simulink model "BEV_WHR"  (R2023a)
settings: Solver=ode23tb  StartTime=0.0  StopTime=20e3  MaxStep=1  RelTol=1e-3
values from neighbouring files (symbols this model uses):
  mass = 20e3    (= 20000)    [run_BEV_simulations.m]    (also in run_FCHEV_simulations.m)
libraries: component_lib x107, slpidlib x8
(part 1 of 2)
settings Model: Creator=maxjo  LastModifiedBy=maxjo
settings SolverCC: ZeroCrossControl=DisableAll

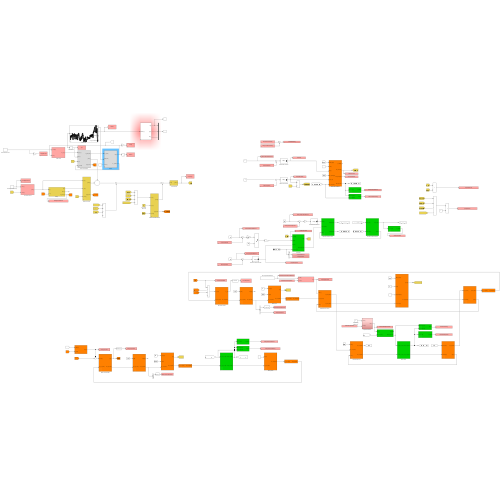
[thumbnail: Simulink's stored preview of the top-level diagram]
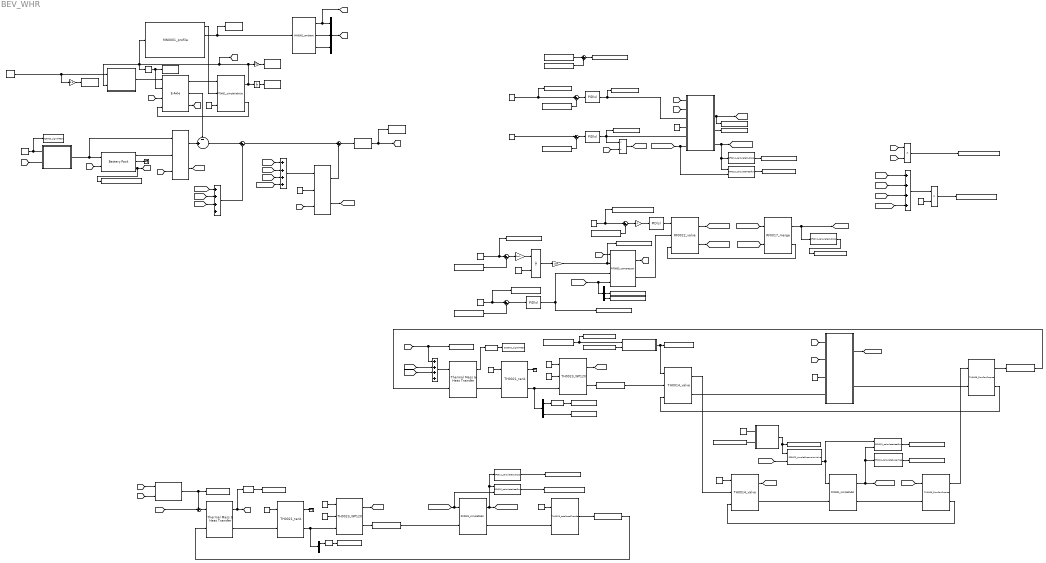
== system BEV_WHR ==
  Add{,1..3} (4 alike) : Sum  Inputs=++++
  Add Constant{,1..3} (4 alike) : Bias  Bias=-273.15  SaturateOnIntegerOverflow=off
  Battery : component_lib/Battery Pack  SOC_0=0.9  Nx=250  Ny=180
  Battery Heater : component_lib/Thermal Systems/TH0015_totalHeatTransfer  T_max=273+100  T_min=273
  Battery Thermal Mass : component_lib/Thermal Mass & Heat Transfer  n=100  d=10e-3  L=4  m=250 * 180 * 0.048  cp=1040  T_0=273 + 20
  Bus Voltage Control : Subsystem
  Bus Voltage Reference [V] : Constant  Value=700
  Cabin Airflow Controller : slpidlib/PID Controller  Controller=PID  Form=Parallel  TimeDomain=Continuous-time  UseExternalTs=off  SampleTime=-1  IntegratorMethod=Forward Euler  FilterMethod=Forward Euler  ControllerParametersSource=internal  P=1  I=1e-1  UseKiTs=off  D=0  N=100  UseFilter=on  TunerSelectOption=Transfer Function Based (PID Tuner App)  InitialConditionSource=internal  InitialConditionForIntegrator=0.5  InitialConditionForFilter=0  DifferentiatorICPrevScaledInput=0  ExternalReset=none  TrackingMode=off  Kt=1  LimitOutput=on  SatLimitsSource=internal  UpperSaturationLimit=1  LowerSaturationLimit=0  LinearizeAsGain=on  AntiWindupMode=clamping  Kb=1  LimitIntegrator=off  UpperIntegratorSaturationLimit=inf  LowerIntegratorSaturationLimit=-inf  POutMin=[]  POutMax=[]  IOutMin=[]  IOutMax=[]  DOutMin=[]  DOutMax=[]  NOutMin=[]  NOutMax=[]  SumOutMin=[]  SumOutMax=[]  SaturationOutMin=[]  SaturationOutMax=[]  PParamMin=[]  PParamMax=[]  IParamMin=[]  IParamMax=[]  DParamMin=[]  DParamMax=[]  NParamMin=[]  NParamMax=[]  KbParamMin=[]  KbParamMax=[]  KtParamMin=[]  KtParamMax=[]  KbOutMin=[]  KbOutMax=[]  KtOutMin=[]  KtOutMax=[]  IntegratorOutMin=[]  IntegratorOutMax=[]  FilterOutMin=[]  FilterOutMax=[]  SumI1OutMin=[]  SumI1OutMax=[]  SumI2OutMin=[]  SumI2OutMax=[]  SumI3OutMin=[]  SumI3OutMax=[]  SumI4OutMin=[]  SumI4OutMax=[]  SumDOutMin=[]  SumDOutMax=[]  DifferentiatorOutMin=[]  DifferentiatorOutMax=[]  FilterDiffOutCoefMin=[]  FilterDiffOutCoefMax=[]  ReciprocalOutMin=[]  ReciprocalOutMax=[]  SumDenOutMin=[]  SumDenOutMax=[]  SumNumOutMin=[]  SumNumOutMax=[]  DivideOutMin=[]  DivideOutMax=[]  UdiffTsProdOutMin=[]  UdiffTsProdOutMax=[]  NTsProdOutMin=[]  NTsProdOutMax=[]  UintegralTsProdOutMin=[]  UintegralTsProdOutMax=[]  UngainTsProdOutMin=[]  UngainTsProdOutMax=[]  ClampingZeroOutDataTypeStr=Inherit: Inherit via back propagation  ClampingZeroOutMin=[]  ClampingZeroOutMax=[]  FilterDenConstantOutDataTypeStr=Inherit: Inherit via back propagation  FilterDenConstantOutMin=[]  FilterDenConstantOutMax=[]  PCopyOutDataTypeStr=Inherit: Inherit via back propagation  PCopyOutMin=[]  PCopyOutMax=[]  NCopyOutDataTypeStr=Inherit: Inherit via back propagation  NCopyOutMin=[]  NCopyOutMax=[]  IntegratorContinuousStateAttributes=''  IntegratorStateMustResolveToSignalObject=off  IntegratorRTWStateStorageClass=Auto  FilterContinuousStateAttributes=''  FilterStateMustResolveToSignalObject=off  FilterRTWStateStorageClass=Auto  ParallelPVariant=InternalParameters  IdealPVariant=Disabled  IVariant=InternalParameters  DVariant=InternalParameters  IntegratorVariant=Continuous  SatVariant=Enabled  AWVariant=ContClampingParallel  PCopyVariant=Disabled  TRVariant=Disabled  FdbkBlocksVariant=Forward  IdealPFdbkVariant=Disabled  SatFdbkVariant=Disabled  DerivativeFilterVariant=ContFilter  NVariant=InternalParameters  NCopyVariant=Disabled  FilterICVariant=InternalICsFilter  IntegratorICVariant=InternalICs  ExternalResetVariant=Disabled  TRSumVariant=Passthrough  SumFdbkVariant=Disabled  SumVariant=Sum_PID  TsampFilterVariant=InternalTs  TsampNgainVariant=Passthrough  TsampIntegralVariant=Disabled_SignalSpec  ExternalSaturationOutDataTypeStr=Inherit: Same as second input
  Cabin with Condenser : Subsystem
  Chassi : component_lib/Powertrain/PT0001_simpleVehicle  m=mass  r_w=0.5  A_f=10  C_d=0.5  rho_air=1.225  c_r0=0.0060  c_r1=2.3e-7  gain=600  v0=75/3.6  x0=0
  Chiller Bypass Valve : component_lib/Thermal Systems/TH0014_valve  d=10e-2  dr=5e-2  C_d=0.9
  Compressor : component_lib/Thermal Systems/RF0003_compressor  V_disp=0.00017  N_ref=2000  t_c=1  W0=0
  Compressor Speed Controller : slpidlib/PID Controller  Controller=PID  Form=Parallel  TimeDomain=Continuous-time  UseExternalTs=off  SampleTime=-1  IntegratorMethod=Forward Euler  FilterMethod=Forward Euler  ControllerParametersSource=internal  P=1e2  I=1e1  UseKiTs=off  D=0  N=100  UseFilter=on  TunerSelectOption=Transfer Function Based (PID Tuner App)  InitialConditionSource=internal  InitialConditionForIntegrator=2000  InitialConditionForFilter=2000  DifferentiatorICPrevScaledInput=0  ExternalReset=none  TrackingMode=off  Kt=1  LimitOutput=on  SatLimitsSource=internal  UpperSaturationLimit=5000  LowerSaturationLimit=500  LinearizeAsGain=on  AntiWindupMode=clamping  Kb=1  LimitIntegrator=off  UpperIntegratorSaturationLimit=inf  LowerIntegratorSaturationLimit=-inf  POutMin=[]  POutMax=[]  IOutMin=[]  IOutMax=[]  DOutMin=[]  DOutMax=[]  NOutMin=[]  NOutMax=[]  SumOutMin=[]  SumOutMax=[]  SaturationOutMin=[]  SaturationOutMax=[]  PParamMin=[]  PParamMax=[]  IParamMin=[]  IParamMax=[]  DParamMin=[]  DParamMax=[]  NParamMin=[]  NParamMax=[]  KbParamMin=[]  KbParamMax=[]  KtParamMin=[]  KtParamMax=[]  KbOutMin=[]  KbOutMax=[]  KtOutMin=[]  KtOutMax=[]  IntegratorOutMin=[]  IntegratorOutMax=[]  FilterOutMin=[]  FilterOutMax=[]  SumI1OutMin=[]  SumI1OutMax=[]  SumI2OutMin=[]  SumI2OutMax=[]  SumI3OutMin=[]  SumI3OutMax=[]  SumI4OutMin=[]  SumI4OutMax=[]  SumDOutMin=[]  SumDOutMax=[]  DifferentiatorOutMin=[]  DifferentiatorOutMax=[]  FilterDiffOutCoefMin=[]  FilterDiffOutCoefMax=[]  ReciprocalOutMin=[]  ReciprocalOutMax=[]  SumDenOutMin=[]  SumDenOutMax=[]  SumNumOutMin=[]  SumNumOutMax=[]  DivideOutMin=[]  DivideOutMax=[]  UdiffTsProdOutMin=[]  UdiffTsProdOutMax=[]  NTsProdOutMin=[]  NTsProdOutMax=[]  UintegralTsProdOutMin=[]  UintegralTsProdOutMax=[]  UngainTsProdOutMin=[]  UngainTsProdOutMax=[]  ClampingZeroOutDataTypeStr=Inherit: Inherit via back propagation  ClampingZeroOutMin=[]  ClampingZeroOutMax=[]  FilterDenConstantOutDataTypeStr=Inherit: Inherit via back propagation  FilterDenConstantOutMin=[]  FilterDenConstantOutMax=[]  PCopyOutDataTypeStr=Inherit: Inherit via back propagation  PCopyOutMin=[]  PCopyOutMax=[]  NCopyOutDataTypeStr=Inherit: Inherit via back propagation  NCopyOutMin=[]  NCopyOutMax=[]  IntegratorContinuousStateAttributes=''  IntegratorStateMustResolveToSignalObject=off  IntegratorRTWStateStorageClass=Auto  FilterContinuousStateAttributes=''  FilterStateMustResolveToSignalObject=off  FilterRTWStateStorageClass=Auto  ParallelPVariant=InternalParameters  IdealPVariant=Disabled  IVariant=InternalParameters  DVariant=InternalParameters  IntegratorVariant=Continuous  SatVariant=Enabled  AWVariant=ContClampingParallel  PCopyVariant=Disabled  TRVariant=Disabled  FdbkBlocksVariant=Forward  IdealPFdbkVariant=Disabled  SatFdbkVariant=Disabled  DerivativeFilterVariant=ContFilter  NVariant=InternalParameters  NCopyVariant=Disabled  FilterICVariant=InternalICsFilter  IntegratorICVariant=InternalICs  ExternalResetVariant=Disabled  TRSumVariant=Passthrough  SumFdbkVariant=Disabled  SumVariant=Sum_PID  TsampFilterVariant=InternalTs  TsampNgainVariant=Passthrough  TsampIntegralVariant=Disabled_SignalSpec  ExternalSaturationOutDataTypeStr=Inherit: Same as second input
  Condenser Valve Controller : slpidlib/PID Controller  Controller=PID  Form=Parallel  TimeDomain=Continuous-time  UseExternalTs=off  SampleTime=-1  IntegratorMethod=Forward Euler  FilterMethod=Forward Euler  ControllerParametersSource=internal  P=1e-1  I=1e-2  UseKiTs=off  D=0  N=100  UseFilter=on  TunerSelectOption=Transfer Function Based (PID Tuner App)  InitialConditionSource=internal  InitialConditionForIntegrator=0.5  InitialConditionForFilter=0.5  DifferentiatorICPrevScaledInput=0  ExternalReset=none  TrackingMode=off  Kt=1  LimitOutput=on  SatLimitsSource=internal  UpperSaturationLimit=1  LowerSaturationLimit=0  LinearizeAsGain=on  AntiWindupMode=clamping  Kb=1  LimitIntegrator=off  UpperIntegratorSaturationLimit=inf  LowerIntegratorSaturationLimit=-inf  POutMin=[]  POutMax=[]  IOutMin=[]  IOutMax=[]  DOutMin=[]  DOutMax=[]  NOutMin=[]  NOutMax=[]  SumOutMin=[]  SumOutMax=[]  SaturationOutMin=[]  SaturationOutMax=[]  PParamMin=[]  PParamMax=[]  IParamMin=[]  IParamMax=[]  DParamMin=[]  DParamMax=[]  NParamMin=[]  NParamMax=[]  KbParamMin=[]  KbParamMax=[]  KtParamMin=[]  KtParamMax=[]  KbOutMin=[]  KbOutMax=[]  KtOutMin=[]  KtOutMax=[]  IntegratorOutMin=[]  IntegratorOutMax=[]  FilterOutMin=[]  FilterOutMax=[]  SumI1OutMin=[]  SumI1OutMax=[]  SumI2OutMin=[]  SumI2OutMax=[]  SumI3OutMin=[]  SumI3OutMax=[]  SumI4OutMin=[]  SumI4OutMax=[]  SumDOutMin=[]  SumDOutMax=[]  DifferentiatorOutMin=[]  DifferentiatorOutMax=[]  FilterDiffOutCoefMin=[]  FilterDiffOutCoefMax=[]  ReciprocalOutMin=[]  ReciprocalOutMax=[]  SumDenOutMin=[]  SumDenOutMax=[]  SumNumOutMin=[]  SumNumOutMax=[]  DivideOutMin=[]  DivideOutMax=[]  UdiffTsProdOutMin=[]  UdiffTsProdOutMax=[]  NTsProdOutMin=[]  NTsProdOutMax=[]  UintegralTsProdOutMin=[]  UintegralTsProdOutMax=[]  UngainTsProdOutMin=[]  UngainTsProdOutMax=[]  ClampingZeroOutDataTypeStr=Inherit: Inherit via back propagation  ClampingZeroOutMin=[]  ClampingZeroOutMax=[]  FilterDenConstantOutDataTypeStr=Inherit: Inherit via back propagation  FilterDenConstantOutMin=[]  FilterDenConstantOutMax=[]  PCopyOutDataTypeStr=Inherit: Inherit via back propagation  PCopyOutMin=[]  PCopyOutMax=[]  NCopyOutDataTypeStr=Inherit: Inherit via back propagation  NCopyOutMin=[]  NCopyOutMax=[]  IntegratorContinuousStateAttributes=''  IntegratorStateMustResolveToSignalObject=off  IntegratorRTWStateStorageClass=Auto  FilterContinuousStateAttributes=''  FilterStateMustResolveToSignalObject=off  FilterRTWStateStorageClass=Auto  ParallelPVariant=InternalParameters  IdealPVariant=Disabled  IVariant=InternalParameters  DVariant=InternalParameters  IntegratorVariant=Continuous  SatVariant=Enabled  AWVariant=ContClampingParallel  PCopyVariant=Disabled  TRVariant=Disabled  FdbkBlocksVariant=Forward  IdealPFdbkVariant=Disabled  SatFdbkVariant=Disabled  DerivativeFilterVariant=ContFilter  NVariant=InternalParameters  NCopyVariant=Disabled  FilterICVariant=InternalICsFilter  IntegratorICVariant=InternalICs  ExternalResetVariant=Disabled  TRSumVariant=Passthrough  SumFdbkVariant=Disabled  SumVariant=Sum_PID  TsampFilterVariant=InternalTs  TsampNgainVariant=Passthrough  TsampIntegralVariant=Disabled_SignalSpec  ExternalSaturationOutDataTypeStr=Inherit: Same as second input
  Constant : Constant  Value=2e5
  Constant1 : Constant  Value=0
  Constant10 : Constant  Value=0.85
  Constant11 : Constant  Value=0
  Constant12 : Constant  Value=2e5
  Constant13 : Constant  Value=3000
  Constant14 : Constant  Value=24
  Constant15 : Constant  Value=24
  Constant16 : Constant  Value=0
  Constant2 : Constant  Value=3000
  Constant23 : Constant  Value=10
  Constant24 : Constant  Value=10
  Constant3 : Constant  Value=24
  Constant4 : Constant  Value=23
  Constant6 : Constant  Value=0.1
  Constant7 : Constant  Value=4000
  Constant8 : Constant  Value=20
  Constant9 : Constant  Value=22.5
  DC/DC - Low level converter : component_lib/Electrochemistry/EL0008_dcdcConverter  eta_up=0.98  eta_down=0.98
  DC/DC Converter : component_lib/Electrochemistry/EL0008_dcdcConverter  eta_up=0.99  eta_down=0.99
  Demux : Demux  Outputs=3
  Demux1 : Demux  Outputs=3
  Demux2 : Demux  Outputs=3
  Divide : Product  Inputs=*/
  Gain : Gain  Gain=3.6
  Gain1 : Gain  Gain=3.6
  Gain2 : Gain  Gain=-1
  Gain4 : Gain  Gain=1e5
  Gain5 : Gain  Gain=1e-1
  Gear selector : Relay  OnSwitchValue=22  OffSwitchValue=21.5  OnOutputValue=4  OffOutputValue=3
  Heat Pump Controller : slpidlib/PID Controller  Controller=PID  Form=Parallel  TimeDomain=Continuous-time  UseExternalTs=off  SampleTime=-1  IntegratorMethod=Forward Euler  FilterMethod=Forward Euler  ControllerParametersSource=internal  P=1e2  I=1e1  UseKiTs=off  D=0  N=100  UseFilter=on  TunerSelectOption=Transfer Function Based (PID Tuner App)  InitialConditionSource=internal  InitialConditionForIntegrator=1500  InitialConditionForFilter=0  DifferentiatorICPrevScaledInput=0  ExternalReset=none  TrackingMode=off  Kt=1  LimitOutput=on  SatLimitsSource=internal  UpperSaturationLimit=inf  LowerSaturationLimit=0  LinearizeAsGain=on  AntiWindupMode=clamping  Kb=1  LimitIntegrator=off  UpperIntegratorSaturationLimit=inf  LowerIntegratorSaturationLimit=-inf  POutMin=[]  POutMax=[]  IOutMin=[]  IOutMax=[]  DOutMin=[]  DOutMax=[]  NOutMin=[]  NOutMax=[]  SumOutMin=[]  SumOutMax=[]  SaturationOutMin=[]  SaturationOutMax=[]  PParamMin=[]  PParamMax=[]  IParamMin=[]  IParamMax=[]  DParamMin=[]  DParamMax=[]  NParamMin=[]  NParamMax=[]  KbParamMin=[]  KbParamMax=[]  KtParamMin=[]  KtParamMax=[]  KbOutMin=[]  KbOutMax=[]  KtOutMin=[]  KtOutMax=[]  IntegratorOutMin=[]  IntegratorOutMax=[]  FilterOutMin=[]  FilterOutMax=[]  SumI1OutMin=[]  SumI1OutMax=[]  SumI2OutMin=[]  SumI2OutMax=[]  SumI3OutMin=[]  SumI3OutMax=[]  SumI4OutMin=[]  SumI4OutMax=[]  SumDOutMin=[]  SumDOutMax=[]  DifferentiatorOutMin=[]  DifferentiatorOutMax=[]  FilterDiffOutCoefMin=[]  FilterDiffOutCoefMax=[]  ReciprocalOutMin=[]  ReciprocalOutMax=[]  SumDenOutMin=[]  SumDenOutMax=[]  SumNumOutMin=[]  SumNumOutMax=[]  DivideOutMin=[]  DivideOutMax=[]  UdiffTsProdOutMin=[]  UdiffTsProdOutMax=[]  NTsProdOutMin=[]  NTsProdOutMax=[]  UintegralTsProdOutMin=[]  UintegralTsProdOutMax=[]  UngainTsProdOutMin=[]  UngainTsProdOutMax=[]  ClampingZeroOutDataTypeStr=Inherit: Inherit via back propagation  ClampingZeroOutMin=[]  ClampingZeroOutMax=[]  FilterDenConstantOutDataTypeStr=Inherit: Inherit via back propagation  FilterDenConstantOutMin=[]  FilterDenConstantOutMax=[]  PCopyOutDataTypeStr=Inherit: Inherit via back propagation  PCopyOutMin=[]  PCopyOutMax=[]  NCopyOutDataTypeStr=Inherit: Inherit via back propagation  NCopyOutMin=[]  NCopyOutMax=[]  IntegratorContinuousStateAttributes=''  IntegratorStateMustResolveToSignalObject=off  IntegratorRTWStateStorageClass=Auto  FilterContinuousStateAttributes=''  FilterStateMustResolveToSignalObject=off  FilterRTWStateStorageClass=Auto  ParallelPVariant=InternalParameters  IdealPVariant=Disabled  IVariant=InternalParameters  DVariant=InternalParameters  IntegratorVariant=Continuous  SatVariant=Enabled  AWVariant=ContClampingParallel  PCopyVariant=Disabled  TRVariant=Disabled  FdbkBlocksVariant=Forward  IdealPFdbkVariant=Disabled  SatFdbkVariant=Disabled  DerivativeFilterVariant=ContFilter  NVariant=InternalParameters  NCopyVariant=Disabled  FilterICVariant=InternalICsFilter  IntegratorICVariant=InternalICs  ExternalResetVariant=Disabled  TRSumVariant=Passthrough  SumFdbkVariant=Disabled  SumVariant=Sum_PID  TsampFilterVariant=InternalTs  TsampNgainVariant=Passthrough  TsampIntegralVariant=Disabled_SignalSpec  ExternalSaturationOutDataTypeStr=Inherit: Same as second input
  High Side Condenser Merge : component_lib/Thermal Systems/RF0017_merge  V=1e-3
  High Side Condenser Valve : component_lib/Thermal Systems/RF0022_valve  d=16e-3  dr=8e-3  C_d=0.9
  Integrator : Integrator
  Integrator1 : Integrator  InitialConditionSource=external  LimitOutput=on  UpperSaturationLimit=20  LowerSaturationLimit=7
  Low Voltage Bus Level : Constant  Value=24
  MN0002_ambient : component_lib/Mission/MN0002_ambient  p_0=1.01e5  T_0=T_amb  RH_0=0.2
  Motor Chiller : component_lib/Thermal Systems/RF0021_simplePHEX  N_ch=10  L=180e-3  B=65e-3  H=2e-3  t=0.3e-3  D_h=2.61e-3
  Motor Heat Transfer : component_lib/Thermal Mass & Heat Transfer  n=100*4  d=10e-3  L=0.6  m=400  cp=420  T_0=273 + 70
  Motor Temperature Reference : Constant  Value=60
  Motor and Gearbox : component_lib/E-Axle  n=4  V_nom=700
  Mux : Mux  Inputs=3
  Product1 : Product
  Product2 : Product
  RF0010_calculateSuperHeat1 : component_lib/Thermal Systems/RF0010_calculateSuperHeat
  RF0011_calculateSubCool : component_lib/Thermal Systems/RF0011_calculateSubCool
  RF0011_calculateSubCool1 : component_lib/Thermal Systems/RF0011_calculateSubCool
  RF0011_calculateSubCool2 : component_lib/Thermal Systems/RF0011_calculateSubCool
  RF0013_calculateHeatflow : component_lib/Thermal Systems/RF0013_calculateHeatflow
  RF0013_calculateHeatflow1 : component_lib/Thermal Systems/RF0013_calculateHeatflow
  RF0013_calculateHeatflow3 : component_lib/Thermal Systems/RF0013_calculateHeatflow
  RF0021_simplePHEX : component_lib/Thermal Systems/RF0021_simplePHEX  N_ch=10  L=180e-3  B=65e-3  H=2e-3  t=0.3e-3  D_h=2.61e-3
  RF0022_simpleExpansionValve1 : component_lib/Thermal Systems/RF0022_simpleExpansionValve  D=4*1.8e-3  p_min=100e3  C=0.3
  "Radiator " : Subsystem
  Radiator Bypass Valve1 : component_lib/Thermal Systems/TH0014_valve  d=10e-2  dr=5e-2  C_d=0.9
  Road Profile : component_lib/Mission/MN0001_profile  profile=Sodertalje_Norrkoping.mat  x0=0  N_lookahead=100
  SC0002_signalRead : component_lib/Data & Control/SC0002_signalRead  SigName=velocity
  SC0002_signalRead1 : component_lib/Data & Control/SC0002_signalRead  SigName=gear
  SC0002_signalRead10 : component_lib/Data & Control/SC0002_signalRead  SigName=cabinCondenserHeating
  SC0002_signalRead11 : component_lib/Data & Control/SC0002_signalRead  SigName=motorGeneratedHeat
  SC0002_signalRead12 : component_lib/Data & Control/SC0002_signalRead  SigName=batteryGeneratedHeat
  SC0002_signalRead13 : component_lib/Data & Control/SC0002_signalRead  SigName=cabinFreshAirFlowReference
  SC0002_signalRead14 : component_lib/Data & Control/SC0002_signalRead  SigName=cabinFlap
  SC0002_signalRead15 : component_lib/Data & Control/SC0002_signalRead  SigName=evaporatorPressure
  SC0002_signalRead16 : component_lib/Data & Control/SC0002_signalRead  SigName=batteryConvection
  SC0002_signalRead17 : component_lib/Data & Control/SC0002_signalRead  SigName=batteryCoolantTemperature
  SC0002_signalRead18 : component_lib/Data & Control/SC0002_signalRead  SigName=radiatorCoolantTemperature
  SC0002_signalRead19 : component_lib/Data & Control/SC0002_signalRead  SigName=radiatorCoolantFlow
  SC0002_signalRead2 : component_lib/Data & Control/SC0002_signalRead  SigName=altitude
  SC0002_signalRead20 : component_lib/Data & Control/SC0002_signalRead  SigName=compressorPower
  SC0002_signalRead21 : component_lib/Data & Control/SC0002_signalRead  SigName=motorChillerExpansionValve
  SC0002_signalRead22 : component_lib/Data & Control/SC0002_signalRead  SigName=batteryTemperature
  SC0002_signalRead23 : component_lib/Data & Control/SC0002_signalRead  SigName=cabinHeaterPower
  SC0002_signalRead24 : component_lib/Data & Control/SC0002_signalRead  SigName=batteryCondenserHeating
  SC0002_signalRead25 : component_lib/Data & Control/SC0002_signalRead  SigName=motorTemperature
  SC0002_signalRead26 : component_lib/Data & Control/SC0002_signalRead  SigName=radiatorBypassValve
  SC0002_signalRead27 : component_lib/Data & Control/SC0002_signalRead  SigName=radiatorCoolantTemperatureReference
  SC0002_signalRead28 : component_lib/Data & Control/SC0002_signalRead  SigName=batteryCondenserSubcool
  SC0002_signalRead29 : component_lib/Data & Control/SC0002_signalRead  SigName=cabinFanCurrent
  SC0002_signalRead3 : component_lib/Data & Control/SC0002_signalRead  SigName=velocityReference
  SC0002_signalRead30 : component_lib/Data & Control/SC0002_signalRead  SigName=pumpfanPower
  SC0002_signalRead32 : component_lib/Data & Control/SC0002_signalRead  SigName=batteryTemperatureReference
  SC0002_signalRead33 : component_lib/Data & Control/SC0002_signalRead  SigName=condenserSubcool
  SC0002_signalRead34 : component_lib/Data & Control/SC0002_signalRead  SigName=compressorFlow
  SC0002_signalRead35 : component_lib/Data & Control/SC0002_signalRead  SigName=condenserPressure
  SC0002_signalRead36 : component_lib/Data & Control/SC0002_signalRead  SigName=compressorSpeed
  SC0002_signalRead37 : component_lib/Data & Control/SC0002_signalRead  SigName=cabinTemperatureReference
  SC0002_signalRead38 : component_lib/Data & Control/SC0002_signalRead  SigName=motorChillerSuperheat
  SC0002_signalRead39 : component_lib/Data & Control/SC0002_signalRead  SigName=motorChillerHeating
  SC0002_signalRead4 : component_lib/Data & Control/SC0002_signalRead  SigName=busVoltage
  SC0002_signalRead43 : component_lib/Data & Control/SC0002_signalRead  SigName=condenserSubcoolReference
  SC0002_signalRead5 : component_lib/Data & Control/SC0002_signalRead  SigName=distance
  SC0002_signalRead6 : component_lib/Data & Control/SC0002_signalRead  SigName=busVoltageReference
  SC0002_signalRead7 : component_lib/Data & Control/SC0002_signalRead  SigName=cabinFreshAirFlow
  SC0002_signalRead8 : component_lib/Data & Control/SC0002_signalRead  SigName=condenserHeating
  SC0002_signalRead9 : component_lib/Data & Control/SC0002_signalRead  SigName=cabinCondenserSubcool
  SC0003_signalWrite1 : component_lib/Data & Control/SC0003_signalWrite  SigName=cabinFreshAirFlow
  SC0003_signalWrite2 : component_lib/Data & Control/SC0003_signalWrite  SigName=cabinCondenserHeating
  SC0003_signalWrite3 : component_lib/Data & Control/SC0003_signalWrite  SigName=cabinTemperature
  SC0003_signalWrite4 : component_lib/Data & Control/SC0003_signalWrite  SigName=radiatorCoolantTemperature
  SC0003_signalWrite5 : component_lib/Data & Control/SC0003_signalWrite  SigName=condenserSubcool
  SC0003_signalWrite6 : component_lib/Data & Control/SC0003_signalWrite  SigName=batteryCoolantTemperature
  SC0003_signalWrite7 : component_lib/Data & Control/SC0003_signalWrite  SigName=batteryCondenserHeating
  SC0003_signalWrite8 : component_lib/Data & Control/SC0003_signalWrite  SigName=cabinTemperature
  SC0003_signalWrite9 : component_lib/Data & Control/SC0003_signalWrite  SigName=motorChillerSuperheat
  Speed control : Subsystem
  Speed reference [m/s] : Constant  Value=80/3.6
  Subsystem2 : Subsystem
  Sum : Sum  Inputs=-+|
  Sum{1..2,5..8,11} (7 alike) : Sum  Inputs=|+-
  Sum3 : Sum  Inputs=|++
  Sum4 : Sum  Inputs=++|
  Super Capacitor : component_lib/Electrochemistry/EL0010_superCapacitor  C=100  V_bus0=700
  Superheat Control1 : Subsystem
  Superheating Reference1 : Constant  Value=5
  TH0006_flowConfluence : component_lib/Thermal Systems/TH0006_flowConfluence  gain=0.01
  TH0006_flowConfluence2 : component_lib/Thermal Systems/TH0006_flowConfluence  gain=0.01
  TH0011_pipe : component_lib/Thermal Systems/TH0011_pipe  d=19e-3  L=5  e=0.006e-3  T_0=273 + 20
  TH0011_pipe1 : component_lib/Thermal Systems/TH0011_pipe  d=19e-3  L=2  e=0.006e-3  T_0=273 + 20
  TH0011_pipe2 : component_lib/Thermal Systems/TH0011_pipe  d=19e-3  L=2  e=0.006e-3  T_0=273 + 20
  TH0011_pipe3 : component_lib/Thermal Systems/TH0011_pipe  d=19e-3  L=5  e=0.006e-3  T_0=273 + 20
  TH0021_tank : component_lib/Thermal Systems/TH0021_tank  V=5e-3  T0=273.15 + 20
  TH0021_tank1 : component_lib/Thermal Systems/TH0021_tank  V=5e-3  T0=273.15 + 25
  TH0023_WP1 : component_lib/Thermal Systems/TH0023_WP120  SystemSampleTime=-1  VariantActivationTime=update diagram  Latency=0  AutoFrameSizeCalculation=off
  TH0023_WP120 : component_lib/Thermal Systems/TH0023_WP120  SystemSampleTime=-1  VariantActivationTime=update diagram  Latency=0  AutoFrameSizeCalculation=off
  TH0030_batteryPackConvection : component_lib/Thermal Systems/TH0030_batteryPackConvection  A=2*10  h=8
  Terminator2 : Terminator
  Terminator3 : Terminator
  Terminator4 : Terminator
  wires:
  Speed reference [m/s]/1 -> Speed control/1(v_ref [m/s]), Gain1/1
  Motor and Gearbox/2 -> Sum/1
  Bus Voltage Reference [V]/1 -> Bus Voltage Control/1(V_ref [V]), SC0002_signalRead6/1
  Chassi/1 -> Integrator/1, Gain/1, [v], Speed control/2(v [m/s]), Road Profile/1, Gear selector/1
  Battery/2 -> Terminator2/1
  Motor and Gearbox/1 -> Chassi/1
  DC/DC Converter/1 -> Sum/2
  Road Profile/1 -> Chassi/2
  Road Profile/2 -> MN0002_ambient/1, SC0002_signalRead2/1
  Constant1/1 -> Chassi/3
  [T_bat] -> Battery/2
  Gain/1 -> SC0002_signalRead/1
  Gear selector/1 -> Motor and Gearbox/2, SC0002_signalRead1/1
  Gain1/1 -> SC0002_signalRead3/1
  Chassi/2 -> Motor and Gearbox/4
  Bus Voltage Control/1(I_bat [-]) -> DC/DC Converter/1, Battery/1
  Integrator/1 -> SC0002_signalRead5/1
  Speed control/1(Tq_sig [-]) -> Motor and Gearbox/1
  Super Capacitor/1 -> [V_bus], SC0002_signalRead4/1
  Battery/1 -> DC/DC Converter/2
  Battery/3 -> SC0002_signalRead12/1, [Q_bat]
  Motor and Gearbox/3 -> [Q_em]
  Cabin Airflow Controller/1 -> Cabin with Condenser/3(flap [-]), SC0002_signalRead14/1
  Constant7/1 -> Cabin with Condenser/4(fan_speed [rpm])
  [v] -> Cabin with Condenser/2(v [m/s])
  MN0002_ambient/3 -> Mux/3
  MN0002_ambient/1 -> [T_amb], Mux/1
  MN0002_ambient/2 -> Mux/2
  Mux/1 -> [amb]
  [amb] -> Cabin with Condenser/1(AMB (T,p,RH))
  Cabin with Condenser/3(fresh_flow [kg/s]) -> SC0002_signalRead7/1
  SC0003_signalWrite1/1 -> Sum2/2
  Sum2/1 -> Cabin Airflow Controller/1
  Constant6/1 -> Sum2/1, SC0002_signalRead13/1
  Battery Thermal Mass/1 -> [T_bat], Add Constant/1
  Battery Heater/1 -> TH0011_pipe/1
  Constant/1 -> TH0021_tank/1
  TH0021_tank/2 -> Demux/1, TH0023_WP120/3
  TH0023_WP120/2 -> TH0011_pipe1/1
  Battery Thermal Mass/2 -> TH0021_tank/2
  Constant2/1 -> TH0023_WP120/2
  Constant3/1 -> TH0023_WP120/1
  TH0023_WP120/1 -> [I_batPump]
  TH0021_tank/1 -> Terminator3/1
  Add Constant/1 -> SC0002_signalRead22/1
  [T_bat] -> TH0030_batteryPackConvection/2
  [T_amb] -> TH0030_batteryPackConvection/1
  [Q_bat] -> Sum4/2
  Sum4/1 -> Battery Thermal Mass/1
  TH0030_batteryPackConvection/1 -> SC0002_signalRead16/1, Sum4/1
  TH0011_pipe/1 -> Battery Thermal Mass/2
  Demux/1 -> Add Constant1/1
  Add Constant1/1 -> SC0002_signalRead17/1
  Radiator Bypass Valve1/1 -> Chiller Bypass Valve/2
  TH0006_flowConfluence/1 -> TH0006_flowConfluence2/1
  [amb] -> "Radiator "/1(AMB: (T,p,RH))
  Motor Temperature Reference/1 -> SC0002_signalRead27/1, Subsystem2/1(T_ref [K])
  Subsystem2/1(cv [-]) -> Radiator Bypass Valve1/1, SC0002_signalRead26/1
  SC0003_signalWrite4/1 -> Subsystem2/2(T_em [K])
  Motor Heat Transfer/1 -> Add Constant3/1
  DC/DC Converter/2 -> [Q_HVDCDC]
  TH0023_WP1/2 -> TH0011_pipe2/1
  Add Constant2/1 -> SC0002_signalRead18/1
  Constant12/1 -> TH0021_tank1/1
  Constant14/1 -> TH0023_WP1/1
  TH0021_tank1/1 -> Terminator4/1
  TH0021_tank1/2 -> Demux1/1, TH0023_WP1/3
  TH0023_WP1/1 -> [I_radPump]
  Constant13/1 -> TH0023_WP1/2
  Demux1/1 -> Add Constant2/1
  Motor Heat Transfer/2 -> TH0021_tank1/2
  Add Constant3/1 -> SC0002_signalRead25/1
  TH0006_flowConfluence2/2 -> Radiator Bypass Valve1/3
  [v] -> "Radiator "/2(v [m/s])
  "Radiator "/1(I_fan [A]) -> [I_radFan]
  Demux1/3 -> SC0002_signalRead19/1
  [Q_em] -> SC0002_signalRead11/1, Add/1
  [V_bus] -> DC/DC - Low level converter/3
  Low Voltage Bus Level/1 -> DC/DC - Low level converter/2
  DC/DC - Low level converter/1 -> Sum6/2
  DC/DC - Low level converter/2 -> [Q_LVDCDC]
  Sum6/1 -> Super Capacitor/1
  [V_bus] -> DC/DC Converter/3
  [V_bus] -> Bus Voltage Control/2(V_bus [V])
  [V_bus] -> Motor and Gearbox/3
  Add/1 -> Motor Heat Transfer/1
  [Q_HVDCDC] -> Add/2
  [Q_LVDCDC] -> Add/3
  Sum/1 -> Sum5/1
  Sum5/1 -> Sum6/1
  Add1/1 -> Sum5/2
  [I_cabHeater] -> Add1/1
  [I_batHeater] -> Add1/2
  RF0011_calculateSubCool/1 -> SC0002_signalRead9/1
  Radiator Bypass Valve1/2 -> "Radiator "/4(CL: (T1,p1,W1))
  "Radiator "/2(CL: (T2,p2,W2)) -> TH0006_flowConfluence2/2
  Constant16/1 -> "Radiator "/3(fan_speed [rpm])
  Cabin with Condenser/4(RF: (h2,p2,W2)) -> [RF_CABCOND_OUT], RF0013_calculateHeatflow/1, RF0011_calculateSubCool/1
  Constant9/1 -> Sum7/1
  Sum7/1 -> Heat Pump Controller/1
  SC0003_signalWrite3/1 -> Sum7/2
  Heat Pump Controller/1 -> Divide/1, Cabin with Condenser/5(Q_ptc [J/s]), SC0002_signalRead23/1
  Cabin with Condenser/2(fan_current [A]) -> SC0002_signalRead29/1, [I_cabFan]
  Compressor/2 -> High Side Condenser Valve/2
  Condenser Valve Controller/1 -> High Side Condenser Valve/1
  High Side Condenser Valve/1 -> [RF_CABCOND_IN]
  [RF_CABCOND_OUT] -> High Side Condenser Merge/1
  High Side Condenser Valve/2 -> [RF_BATCOND_IN]
  [RF_BATCOND_OUT] -> High Side Condenser Merge/2
  High Side Condenser Merge/2 -> High Side Condenser Valve/3
  [RF_CHILL_OUT] -> Compressor/4, Demux2/1
  RF0021_simplePHEX/2 -> Battery Heater/2
  TH0011_pipe1/1 -> RF0021_simplePHEX/2
  [RF_BATCOND_IN] -> RF0013_calculateHeatflow1/2, RF0021_simplePHEX/1
  RF0013_calculateHeatflow/1 -> SC0002_signalRead10/1
  [RF_CABCOND_IN] -> Cabin with Condenser/6(RF: (h1,p1,W1)), RF0013_calculateHeatflow/2
  RF0013_calculateHeatflow1/1 -> SC0002_signalRead24/1
  RF0021_simplePHEX/1 -> RF0011_calculateSubCool1/1, RF0013_calculateHeatflow1/1, [RF_BATCOND_OUT]
  RF0011_calculateSubCool1/1 -> SC0002_signalRead28/1
  SC0003_signalWrite6/1 -> Sum1/2
  Constant8/1 -> Sum1/1, SC0002_signalRead32/1
  Sum1/1 -> Gain2/1
  Gain2/1 -> Condenser Valve Controller/1
  Constant11/1 -> Battery Heater/1
  SC0003_signalWrite2/1 -> Sum3/1
  SC0003_signalWrite7/1 -> Sum3/2
  Sum3/1 -> SC0002_signalRead8/1
  RF0011_calculateSubCool2/1 -> SC0002_signalRead33/1
  Demux2/2 -> SC0002_signalRead15/1
  Demux2/3 -> SC0002_signalRead34/1
  [V_bus] -> Compressor/1
  Compressor/1 -> [I_cmp]
  [I_cmp] -> Add1/3
  [V_bus] -> Divide/2
  Divide/1 -> [I_cabHeater]
  Add2/1 -> DC/DC - Low level converter/1
  [I_cabFan] -> Add2/1
  [I_batPump] -> Add2/2
  [I_radPump] -> Add2/3
  TH0011_pipe2/1 -> Radiator Bypass Valve1/2
  Chiller Bypass Valve/1 -> [CL3]
  [CL3] -> TH0006_flowConfluence/1
  TH0011_pipe3/1 -> Motor Heat Transfer/2
  TH0006_flowConfluence/2 -> Chiller Bypass Valve/3
  Motor Chiller/2 -> TH0006_flowConfluence/2
  Chiller Bypass Valve/2 -> Motor Chiller/2
  Constant10/1 -> Chiller Bypass Valve/1
  [RF_CHILL_IN] -> RF0022_simpleExpansionValve1/2
  RF0022_simpleExpansionValve1/2 -> RF0013_calculateHeatflow3/1, Motor Chiller/1
  Superheat Control1/1(EXV [-]) -> RF0022_simpleExpansionValve1/1, SC0002_signalRead21/1
  Superheating Reference1/1 -> Superheat Control1/1(T_ref [K])
  SC0003_signalWrite9/1 -> Superheat Control1/2(T_sup [K])
  RF0013_calculateHeatflow3/1 -> SC0002_signalRead39/1
  RF0010_calculateSuperHeat1/1 -> SC0002_signalRead38/1
  Motor Chiller/1 -> [RF_CHILL_OUT], RF0010_calculateSuperHeat1/1, RF0013_calculateHeatflow3/2
  High Side Condenser Merge/1 -> [RF_CHILL_IN], RF0011_calculateSubCool2/1
  Add3/1 -> Product2/1
  [I_cabFan] -> Add3/1
  Product2/1 -> SC0002_signalRead30/1
  [I_radPump] -> Add3/3
  [V_bus] -> Product1/1
  Product1/1 -> SC0002_signalRead20/1
  [I_cmp] -> Product1/2
  Constant15/1 -> Product2/2
  [I_batPump] -> Add3/2
  [I_radFan] -> Add3/4
  TH0006_flowConfluence2/1 -> TH0011_pipe3/1
  [I_radFan] -> Add2/4
  Gain4/1 -> Compressor/2, SC0002_signalRead35/1
  Constant24/1 -> Integrator1/2
  SC0003_signalWrite5/1 -> Sum11/2
  Integrator1/1 -> Gain4/1
  Constant23/1 -> SC0002_signalRead43/1, Sum11/1
  Gain5/1 -> Integrator1/1
  Sum11/1 -> Gain5/1
  Compressor Speed Controller/1 -> Compressor/3, SC0002_signalRead36/1
  SC0003_signalWrite8/1 -> Sum8/2
  Sum8/1 -> Compressor Speed Controller/1
  Constant4/1 -> SC0002_signalRead37/1, Sum8/1

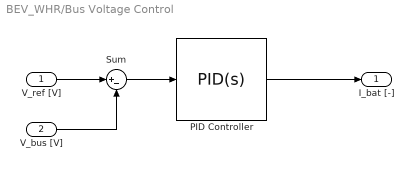
== system BEV_WHR/Bus Voltage Control ==
  V_ref [V] : Inport
  V_bus [V] : Inport  Port=2
  PID Controller : slpidlib/PID Controller  Controller=PID  Form=Parallel  TimeDomain=Continuous-time  UseExternalTs=off  SampleTime=-1  IntegratorMethod=Forward Euler  FilterMethod=Forward Euler  ControllerParametersSource=internal  P=1e2  I=1  UseKiTs=off  D=0  N=100  UseFilter=on  TunerSelectOption=Transfer Function Based (PID Tuner App)  ZeroCross=off  InitialConditionSource=internal  InitialConditionForIntegrator=0  InitialConditionForFilter=0  DifferentiatorICPrevScaledInput=0  ExternalReset=none  TrackingMode=off  Kt=1  LimitOutput=on  SatLimitsSource=internal  UpperSaturationLimit=725*2  LowerSaturationLimit=-725  LinearizeAsGain=on  AntiWindupMode=clamping  Kb=1  LimitIntegrator=off  UpperIntegratorSaturationLimit=inf  LowerIntegratorSaturationLimit=-inf  POutMin=[]  POutMax=[]  IOutMin=[]  IOutMax=[]  DOutMin=[]  DOutMax=[]  NOutMin=[]  NOutMax=[]  SumOutMin=[]  SumOutMax=[]  SaturationOutMin=[]  SaturationOutMax=[]  PParamMin=[]  PParamMax=[]  IParamMin=[]  IParamMax=[]  DParamMin=[]  DParamMax=[]  NParamMin=[]  NParamMax=[]  KbParamMin=[]  KbParamMax=[]  KtParamMin=[]  KtParamMax=[]  KbOutMin=[]  KbOutMax=[]  KtOutMin=[]  KtOutMax=[]  IntegratorOutMin=[]  IntegratorOutMax=[]  FilterOutMin=[]  FilterOutMax=[]  SumI1OutMin=[]  SumI1OutMax=[]  SumI2OutMin=[]  SumI2OutMax=[]  SumI3OutMin=[]  SumI3OutMax=[]  SumI4OutMin=[]  SumI4OutMax=[]  SumDOutMin=[]  SumDOutMax=[]  DifferentiatorOutMin=[]  DifferentiatorOutMax=[]  FilterDiffOutCoefMin=[]  FilterDiffOutCoefMax=[]  ReciprocalOutMin=[]  ReciprocalOutMax=[]  SumDenOutMin=[]  SumDenOutMax=[]  SumNumOutMin=[]  SumNumOutMax=[]  DivideOutMin=[]  DivideOutMax=[]  UdiffTsProdOutMin=[]  UdiffTsProdOutMax=[]  NTsProdOutMin=[]  NTsProdOutMax=[]  UintegralTsProdOutMin=[]  UintegralTsProdOutMax=[]  UngainTsProdOutMin=[]  UngainTsProdOutMax=[]  ClampingZeroOutDataTypeStr=Inherit: Inherit via back propagation  ClampingZeroOutMin=[]  ClampingZeroOutMax=[]  FilterDenConstantOutDataTypeStr=Inherit: Inherit via back propagation  FilterDenConstantOutMin=[]  FilterDenConstantOutMax=[]  PCopyOutDataTypeStr=Inherit: Inherit via back propagation  PCopyOutMin=[]  PCopyOutMax=[]  NCopyOutDataTypeStr=Inherit: Inherit via back propagation  NCopyOutMin=[]  NCopyOutMax=[]  IntegratorContinuousStateAttributes=''  IntegratorStateMustResolveToSignalObject=off  IntegratorRTWStateStorageClass=Auto  FilterContinuousStateAttributes=''  FilterStateMustResolveToSignalObject=off  FilterRTWStateStorageClass=Auto  ParallelPVariant=InternalParameters  IdealPVariant=Disabled  IVariant=InternalParameters  DVariant=InternalParameters  IntegratorVariant=Continuous  SatVariant=Enabled  AWVariant=ContClampingParallel  PCopyVariant=Disabled  TRVariant=Disabled  FdbkBlocksVariant=Forward  IdealPFdbkVariant=Disabled  SatFdbkVariant=Disabled  DerivativeFilterVariant=ContFilter  NVariant=InternalParameters  NCopyVariant=Disabled  FilterICVariant=InternalICsFilter  IntegratorICVariant=InternalICs  ExternalResetVariant=Disabled  TRSumVariant=Passthrough  SumFdbkVariant=Disabled  SumVariant=Sum_PID  TsampFilterVariant=InternalTs  TsampNgainVariant=Passthrough  TsampIntegralVariant=Disabled_SignalSpec  ExternalSaturationOutDataTypeStr=Inherit: Same as second input
  Sum : Sum  Inputs=|+-
  I_bat [-] : Outport
  wires:
  PID Controller/1 -> I_bat [-]/1
  Sum/1 -> PID Controller/1
  V_ref [V]/1 -> Sum/1
  V_bus [V]/1 -> Sum/2

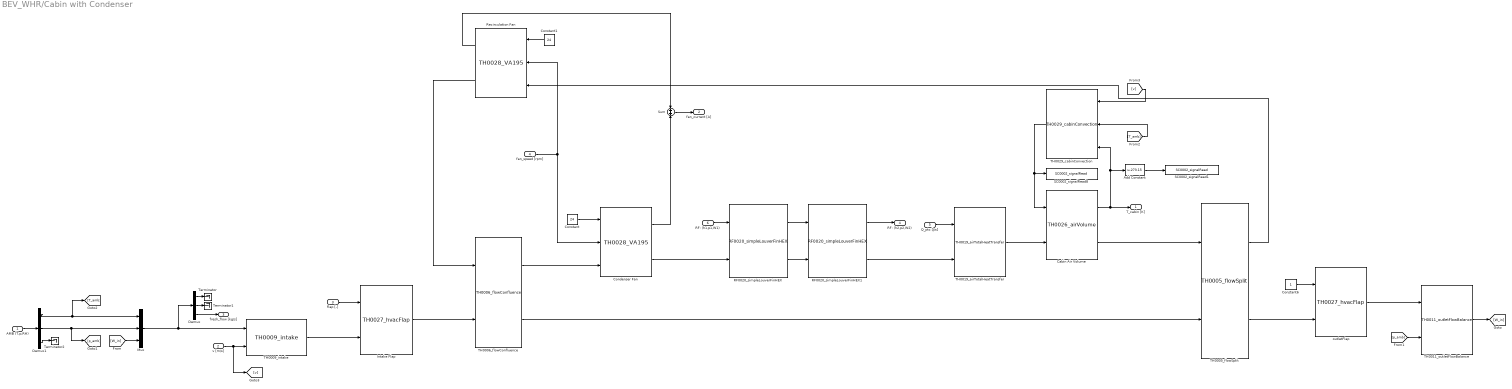
== system BEV_WHR/Cabin with Condenser ==
  AMB (T,p,RH) : Inport
  v [m/s] : Inport  Port=2
  flap [-] : Inport  Port=3
  fan_speed [rpm] : Inport  Port=4
  Q_ptc [J/s] : Inport  Port=5
  RF: (h1,p1,W1) : Inport  Port=6
  Add Constant : Bias  Bias=-273.15  SaturateOnIntegerOverflow=off
  Cabin Air Volume : component_lib/Thermal Systems/TH0026_airVolume  V=4  T0=273.15 + 20
  Condenser Fan : component_lib/Thermal Systems/TH0028_VA195  n=4
      settings: LibrarySourceBlock=component_lib/Thermal Systems/TH0023_WP120
  Constant : Constant  Value=24
  Constant1 : Constant  Value=24
  Constant6 : Constant
  Demux : Demux  Outputs=3
  Demux1 : Demux  Outputs=3
  Intake Flap : component_lib/Thermal Systems/TH0027_hvacFlap  A=0.04  zeta=0.3
  Mux : Mux  Inputs=3
  RF0020_simpleLouverFinHEX : component_lib/Thermal Systems/RF0020_simpleLouverFinHEX  N_tub=20  T_L=0.95*3  T_p=10.15e-3  T_d=16e-3  N_ch=18  a=1.3e-3  b=0.58e-3  L_a=23  F_p=1.4e-3  L_p=1.7e-3  L_l=6.4e-3  H=8.15e-3  d_f=16e-3  F_d=16e-3
  RF0020_simpleLouverFinHEX1 : component_lib/Thermal Systems/RF0020_simpleLouverFinHEX  N_tub=20  T_L=0.95*3  T_p=10.15e-3  T_d=16e-3  N_ch=18  a=1.3e-3  b=0.58e-3  L_a=23  F_p=1.4e-3  L_p=1.7e-3  L_l=6.4e-3  H=8.15e-3  d_f=16e-3  F_d=16e-3
  Recirculation Fan : component_lib/Thermal Systems/TH0028_VA195  n=4
      settings: LibrarySourceBlock=component_lib/Thermal Systems/TH0023_WP120
  SC0002_signalRead1 : component_lib/Data & Control/SC0002_signalRead  SigName=cabinTemperature
  SC0002_signalRead8 : component_lib/Data & Control/SC0002_signalRead  SigName=cabinConvection
  Sum : Sum  Inputs=+|+
  TH0005_flowSplit : component_lib/Thermal Systems/TH0005_flowSplit  SystemSampleTime=-1  VariantActivationTime=update diagram  Latency=0  AutoFrameSizeCalculation=off
  TH0006_flowConfluence : component_lib/Thermal Systems/TH0006_flowConfluence  gain=0.01
  TH0009_intake : component_lib/Thermal Systems/TH0009_intake  zeta=0.1
  TH0011_outletFlowBalance : component_lib/Thermal Systems/TH0011_outletFlowBalance  gain=0.05
  TH0019_airTotalHeatTransfer : component_lib/Thermal Systems/TH0019_airTotalHeatTransfer  T_min=273-40  T_max=273+140
  TH0029_cabinConvection : component_lib/Thermal Systems/TH0029_cabinConvection  A=2
  Terminator : Terminator
  Terminator1 : Terminator
  Terminator2 : Terminator
  outletFlap : component_lib/Thermal Systems/TH0027_hvacFlap  A=0.04  zeta=0.3
  T_cabin [K] : Outport
  fan_current [A] : Outport  Port=2
  fresh_flow [kg/s] : Outport  Port=3
  RF: (h2,p2,W2) : Outport  Port=4
  wires:
  TH0019_airTotalHeatTransfer/1 -> Cabin Air Volume/2
  Q_ptc [J/s]/1 -> TH0019_airTotalHeatTransfer/1
  Add Constant/1 -> SC0002_signalRead1/1
  Demux1/3 -> Terminator2/1
  Demux/2 -> Terminator1/1
  Demux/1 -> Terminator/1
  TH0009_intake/1 -> Intake Flap/2
  Cabin Air Volume/2 -> TH0005_flowSplit/1
  AMB (T,p,RH)/1 -> Demux1/1
  flap [-]/1 -> Intake Flap/1
  Constant/1 -> Condenser Fan/1
  Intake Flap/1 -> TH0006_flowConfluence/2
  [T_amb] -> TH0029_cabinConvection/2
  v [m/s]/1 -> TH0009_intake/2, [v]
  [v] -> TH0029_cabinConvection/1
  Cabin Air Volume/1 -> T_cabin [K]/1, Add Constant/1, TH0029_cabinConvection/3
  TH0005_flowSplit/2 -> outletFlap/2
  TH0006_flowConfluence/2 -> TH0005_flowSplit/2
  TH0029_cabinConvection/1 -> SC0002_signalRead8/1, Cabin Air Volume/1
  TH0005_flowSplit/1 -> Recirculation Fan/3
  Mux/1 -> Demux/1, TH0009_intake/1
  RF: (h1,p1,W1)/1 -> RF0020_simpleLouverFinHEX/1
  Demux1/2 -> [p_amb], Mux/2
  outletFlap/1 -> TH0011_outletFlowBalance/1
  Demux1/1 -> [T_amb], Mux/1
  [W_in] -> Mux/3
  TH0011_outletFlowBalance/1 -> [W_in]
  Constant6/1 -> outletFlap/1
  [p_amb] -> TH0011_outletFlowBalance/2
  Demux/3 -> fresh_flow [kg/s]/1
  TH0006_flowConfluence/1 -> Condenser Fan/3
  Condenser Fan/2 -> RF0020_simpleLouverFinHEX/2
  Recirculation Fan/2 -> TH0006_flowConfluence/1
  Constant1/1 -> Recirculation Fan/1
  fan_speed [rpm]/1 -> Condenser Fan/2, Recirculation Fan/2
  Condenser Fan/1 -> Sum/2
  Sum/1 -> fan_current [A]/1
  Recirculation Fan/1 -> Sum/1
  RF0020_simpleLouverFinHEX/1 -> RF0020_simpleLouverFinHEX1/1
  RF0020_simpleLouverFinHEX/2 -> RF0020_simpleLouverFinHEX1/2
  RF0020_simpleLouverFinHEX1/1 -> RF: (h2,p2,W2)/1
  RF0020_simpleLouverFinHEX1/2 -> TH0019_airTotalHeatTransfer/2

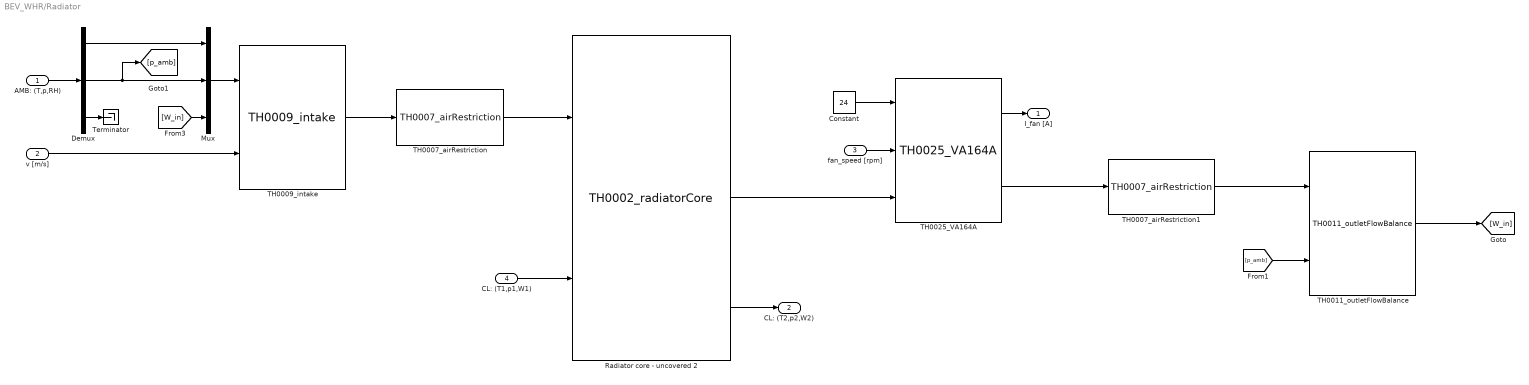
== system BEV_WHR/Radiator  ==
  AMB: (T,p,RH) : Inport
  v [m/s] : Inport  Port=2
  fan_speed [rpm] : Inport  Port=3
  CL: (T1,p1,W1) : Inport  Port=4
  Constant : Constant  Value=24
  Demux : Demux  Outputs=3
  Mux : Mux  Inputs=3
  Radiator core - uncovered 2 : component_lib/Thermal Systems/TH0002_radiatorCore  HtH=1.1  StS=0.95  radmodel=52 mm
  TH0007_airRestriction : component_lib/Thermal Systems/TH0007_airRestriction  A=0.8  zeta=0.3
  TH0007_airRestriction1 : component_lib/Thermal Systems/TH0007_airRestriction  A=1  zeta=2.5
  TH0009_intake : component_lib/Thermal Systems/TH0009_intake  zeta=0.9
  TH0011_outletFlowBalance : component_lib/Thermal Systems/TH0011_outletFlowBalance  gain=0.05
  TH0025_VA164A : component_lib/Thermal Systems/TH0025_VA164A  n=1
      settings: LibrarySourceBlock=component_lib/Thermal Systems/TH0023_WP120
  Terminator : Terminator
  I_fan [A] : Outport
  CL: (T2,p2,W2) : Outport  Port=2
  wires:
  Constant/1 -> TH0025_VA164A/1
  TH0025_VA164A/1 -> I_fan [A]/1
  CL: (T1,p1,W1)/1 -> Radiator core - uncovered 2/2
  Demux/3 -> Terminator/1
  [W_in] -> Mux/3
  TH0011_outletFlowBalance/1 -> [W_in]
  [p_amb] -> TH0011_outletFlowBalance/2
  TH0009_intake/1 -> TH0007_airRestriction/1
  Mux/1 -> TH0009_intake/1
  TH0007_airRestriction1/1 -> TH0011_outletFlowBalance/1
  v [m/s]/1 -> TH0009_intake/2
  fan_speed [rpm]/1 -> TH0025_VA164A/2
  Radiator core - uncovered 2/3 -> CL: (T2,p2,W2)/1
  AMB: (T,p,RH)/1 -> Demux/1
  Demux/1 -> Mux/1
  Demux/2 -> [p_amb], Mux/2
  Radiator core - uncovered 2/2 -> TH0025_VA164A/3
  TH0025_VA164A/2 -> TH0007_airRestriction1/1
  TH0007_airRestriction/1 -> Radiator core - uncovered 2/1

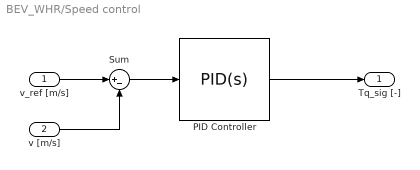
== system BEV_WHR/Speed control ==
  v_ref [m/s] : Inport
  v [m/s] : Inport  Port=2
  PID Controller : slpidlib/PID Controller  Controller=PID  Form=Parallel  TimeDomain=Continuous-time  UseExternalTs=off  SampleTime=-1  IntegratorMethod=Forward Euler  FilterMethod=Forward Euler  ControllerParametersSource=internal  P=10  I=1e-1  UseKiTs=off  D=0  N=100  UseFilter=on  TunerSelectOption=Transfer Function Based (PID Tuner App)  ZeroCross=off  InitialConditionSource=internal  InitialConditionForIntegrator=0  InitialConditionForFilter=0  DifferentiatorICPrevScaledInput=0  ExternalReset=none  TrackingMode=off  Kt=1  LimitOutput=on  SatLimitsSource=internal  UpperSaturationLimit=1  LowerSaturationLimit=-1  LinearizeAsGain=on  AntiWindupMode=clamping  Kb=1  LimitIntegrator=off  UpperIntegratorSaturationLimit=inf  LowerIntegratorSaturationLimit=-inf  POutMin=[]  POutMax=[]  IOutMin=[]  IOutMax=[]  DOutMin=[]  DOutMax=[]  NOutMin=[]  NOutMax=[]  SumOutMin=[]  SumOutMax=[]  SaturationOutMin=[]  SaturationOutMax=[]  PParamMin=[]  PParamMax=[]  IParamMin=[]  IParamMax=[]  DParamMin=[]  DParamMax=[]  NParamMin=[]  NParamMax=[]  KbParamMin=[]  KbParamMax=[]  KtParamMin=[]  KtParamMax=[]  KbOutMin=[]  KbOutMax=[]  KtOutMin=[]  KtOutMax=[]  IntegratorOutMin=[]  IntegratorOutMax=[]  FilterOutMin=[]  FilterOutMax=[]  SumI1OutMin=[]  SumI1OutMax=[]  SumI2OutMin=[]  SumI2OutMax=[]  SumI3OutMin=[]  SumI3OutMax=[]  SumI4OutMin=[]  SumI4OutMax=[]  SumDOutMin=[]  SumDOutMax=[]  DifferentiatorOutMin=[]  DifferentiatorOutMax=[]  FilterDiffOutCoefMin=[]  FilterDiffOutCoefMax=[]  ReciprocalOutMin=[]  ReciprocalOutMax=[]  SumDenOutMin=[]  SumDenOutMax=[]  SumNumOutMin=[]  SumNumOutMax=[]  DivideOutMin=[]  DivideOutMax=[]  UdiffTsProdOutMin=[]  UdiffTsProdOutMax=[]  NTsProdOutMin=[]  NTsProdOutMax=[]  UintegralTsProdOutMin=[]  UintegralTsProdOutMax=[]  UngainTsProdOutMin=[]  UngainTsProdOutMax=[]  ClampingZeroOutDataTypeStr=Inherit: Inherit via back propagation  ClampingZeroOutMin=[]  ClampingZeroOutMax=[]  FilterDenConstantOutDataTypeStr=Inherit: Inherit via back propagation  FilterDenConstantOutMin=[]  FilterDenConstantOutMax=[]  PCopyOutDataTypeStr=Inherit: Inherit via back propagation  PCopyOutMin=[]  PCopyOutMax=[]  NCopyOutDataTypeStr=Inherit: Inherit via back propagation  NCopyOutMin=[]  NCopyOutMax=[]  IntegratorContinuousStateAttributes=''  IntegratorStateMustResolveToSignalObject=off  IntegratorRTWStateStorageClass=Auto  FilterContinuousStateAttributes=''  FilterStateMustResolveToSignalObject=off  FilterRTWStateStorageClass=Auto  ParallelPVariant=InternalParameters  IdealPVariant=Disabled  IVariant=InternalParameters  DVariant=InternalParameters  IntegratorVariant=Continuous  SatVariant=Enabled  AWVariant=ContClampingParallel  PCopyVariant=Disabled  TRVariant=Disabled  FdbkBlocksVariant=Forward  IdealPFdbkVariant=Disabled  SatFdbkVariant=Disabled  DerivativeFilterVariant=ContFilter  NVariant=InternalParameters  NCopyVariant=Disabled  FilterICVariant=InternalICsFilter  IntegratorICVariant=InternalICs  ExternalResetVariant=Disabled  TRSumVariant=Passthrough  SumFdbkVariant=Disabled  SumVariant=Sum_PID  TsampFilterVariant=InternalTs  TsampNgainVariant=Passthrough  TsampIntegralVariant=Disabled_SignalSpec  ExternalSaturationOutDataTypeStr=Inherit: Same as second input
  Sum : Sum  Inputs=|+-
  Tq_sig [-] : Outport
  wires:
  PID Controller/1 -> Tq_sig [-]/1
  Sum/1 -> PID Controller/1
  v_ref [m/s]/1 -> Sum/1
  v [m/s]/1 -> Sum/2

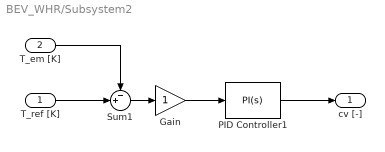
== system BEV_WHR/Subsystem2 ==
  T_ref [K] : Inport
  T_em [K] : Inport  Port=2
  Gain : Gain
  PID Controller1 : slpidlib/PID Controller  Controller=PI  Form=Parallel  TimeDomain=Continuous-time  UseExternalTs=off  SampleTime=-1  IntegratorMethod=Forward Euler  FilterMethod=Forward Euler  ControllerParametersSource=internal  P=1e-1  I=1e-2  UseKiTs=off  D=0  N=100  UseFilter=on  TunerSelectOption=Transfer Function Based (PID Tuner App)  ZeroCross=off  InitialConditionSource=internal  InitialConditionForIntegrator=0.5  InitialConditionForFilter=0.5  DifferentiatorICPrevScaledInput=0  ExternalReset=none  TrackingMode=off  Kt=1  LimitOutput=on  SatLimitsSource=internal  UpperSaturationLimit=0.95  LowerSaturationLimit=0.05  LinearizeAsGain=on  AntiWindupMode=back-calculation  Kb=1  LimitIntegrator=off  UpperIntegratorSaturationLimit=inf  LowerIntegratorSaturationLimit=-inf  POutMin=[]  POutMax=[]  IOutMin=[]  IOutMax=[]  DOutMin=[]  DOutMax=[]  NOutMin=[]  NOutMax=[]  SumOutMin=[]  SumOutMax=[]  SaturationOutMin=[]  SaturationOutMax=[]  PParamMin=[]  PParamMax=[]  IParamMin=[]  IParamMax=[]  DParamMin=[]  DParamMax=[]  NParamMin=[]  NParamMax=[]  KbParamMin=[]  KbParamMax=[]  KtParamMin=[]  KtParamMax=[]  KbOutMin=[]  KbOutMax=[]  KtOutMin=[]  KtOutMax=[]  IntegratorOutMin=[]  IntegratorOutMax=[]  FilterOutMin=[]  FilterOutMax=[]  SumI1OutMin=[]  SumI1OutMax=[]  SumI2OutMin=[]  SumI2OutMax=[]  SumI3OutMin=[]  SumI3OutMax=[]  SumI4OutMin=[]  SumI4OutMax=[]  SumDOutMin=[]  SumDOutMax=[]  DifferentiatorOutMin=[]  DifferentiatorOutMax=[]  FilterDiffOutCoefMin=[]  FilterDiffOutCoefMax=[]  ReciprocalOutMin=[]  ReciprocalOutMax=[]  SumDenOutMin=[]  SumDenOutMax=[]  SumNumOutMin=[]  SumNumOutMax=[]  DivideOutMin=[]  DivideOutMax=[]  UdiffTsProdOutMin=[]  UdiffTsProdOutMax=[]  NTsProdOutMin=[]  NTsProdOutMax=[]  UintegralTsProdOutMin=[]  UintegralTsProdOutMax=[]  UngainTsProdOutMin=[]  UngainTsProdOutMax=[]  ClampingZeroOutDataTypeStr=Inherit: Inherit via back propagation  ClampingZeroOutMin=[]  ClampingZeroOutMax=[]  FilterDenConstantOutDataTypeStr=Inherit: Inherit via back propagation  FilterDenConstantOutMin=[]  FilterDenConstantOutMax=[]  PCopyOutDataTypeStr=Inherit: Inherit via back propagation  PCopyOutMin=[]  PCopyOutMax=[]  NCopyOutDataTypeStr=Inherit: Inherit via back propagation  NCopyOutMin=[]  NCopyOutMax=[]  IntegratorContinuousStateAttributes=''  IntegratorStateMustResolveToSignalObject=off  IntegratorRTWStateStorageClass=Auto  FilterContinuousStateAttributes=''  FilterStateMustResolveToSignalObject=off  FilterRTWStateStorageClass=Auto  ParallelPVariant=InternalParameters  IdealPVariant=Disabled  IVariant=InternalParameters  DVariant=Disabled  IntegratorVariant=Continuous  SatVariant=Enabled  AWVariant=BackCalculation  PCopyVariant=Disabled  TRVariant=Disabled  FdbkBlocksVariant=Forward  IdealPFdbkVariant=Disabled  SatFdbkVariant=Disabled  DerivativeFilterVariant=Disabled  NVariant=Disabled  NCopyVariant=Disabled_SignalSpec  FilterICVariant=Disabled  IntegratorICVariant=InternalICs  ExternalResetVariant=Disabled  TRSumVariant=Passthrough  SumFdbkVariant=Disabled  SumVariant=Sum_PI  TsampFilterVariant=InternalTs  TsampNgainVariant=Passthrough  TsampIntegralVariant=Disabled_SignalSpec  ExternalSaturationOutDataTypeStr=Inherit: Same as second input
  Sum1 : Sum  Inputs=-+|
  cv [-] : Outport
  wires:
  T_em [K]/1 -> Sum1/1
  Gain/1 -> PID Controller1/1
  Sum1/1 -> Gain/1
  PID Controller1/1 -> cv [-]/1
  T_ref [K]/1 -> Sum1/2
